simulink model "DAB"  (R2022a)
settings: Solver=ode23t  StartTime=0.0  StopTime=1.75  RelTol=1e-3
undefined symbols (not defined in the file): Ion, Lithium
libraries: spsIGBTDiodeLib x8, spsSeriesRLCBranchLib x6, spsVoltageMeasurementLib x6, spsCurrentMeasurementLib x4, spsDiodeLib x4, slpidlib x3, spsMosfetLib x2, spsBatteryLib x1, spsFuelCellStackLib x1, spsUniversalBridgeLib x1, spsLinearTransformerLib x1, spsMutualInductanceLib x1
settings Model: Creator=rahul  LastModifiedBy=DELL
settings ModelReferenceCC: EnableRefExpFcnMdlSchedulingChecks=off
settings RTWCC: Description=Generic Real-Time Target  GPUComputeCapability=5.0

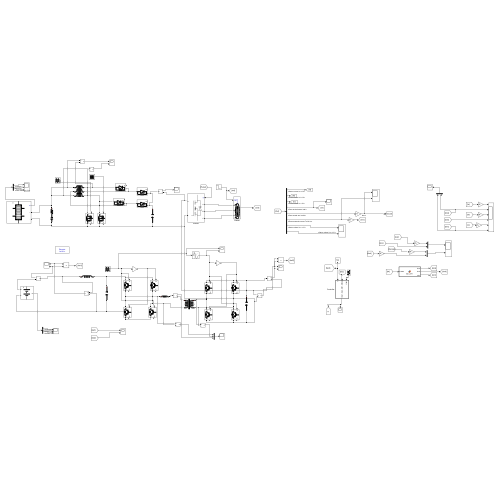
[thumbnail: Simulink's stored preview of the top-level diagram]
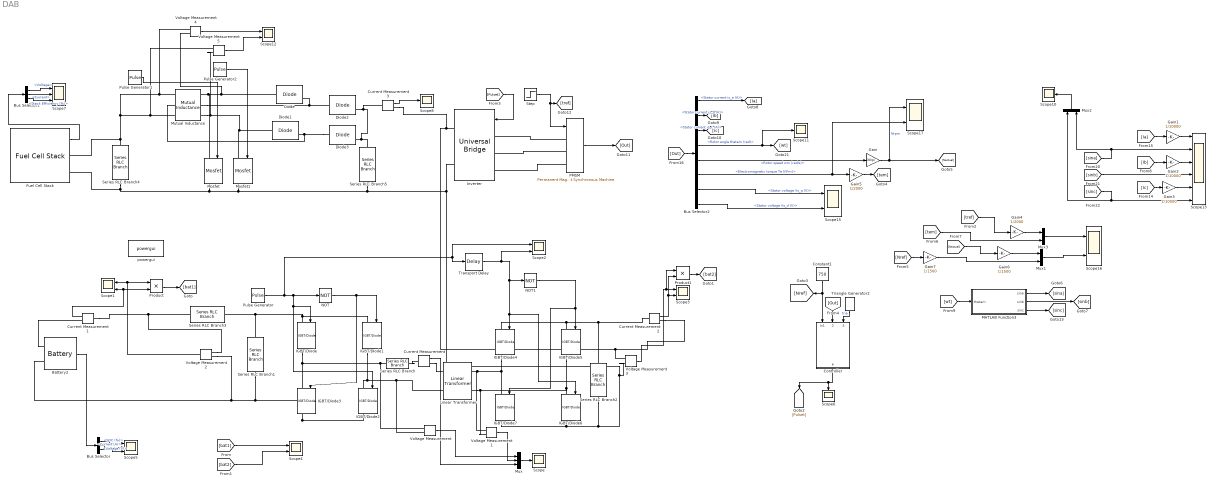
== system DAB ==
  Battery2 : spsBatteryLib/Battery  BatType=Lithium-Ion  ShowTempParam=off  ThermalPreset=no  ShowAgeParam=off  NomV=96  NomQ=26  SOC=50  Batt_Tr=30  PresetModel=on  MaxQ=26  MinV=72  FullV=111.7428  Dis_rate=11.3043  R=0.036923  Normal_OP=23.513  expZone="[103.717      1.277391]"  current=[6.5 13 32.5]  Units=Time  Tci=20  NomT=20  T2=-30  MaxQ2=4.8  FullV2=7.1  Normal_OP2=5.655  expZone2="[6.58           1]"  Rca=0.6  ti=2000  Dp=0  Neq0=0  Tsim=1e6  Ta1=25  Qeol=5.4*0.9  Reol=0.013333*1.2  Char_age=[2.3478, 3]  Dis_age=[2.3478, 10]  N1=1500  N2=10500  N3=1000  N4=1400  Ta2=45  N5=950
  Bus Selector : BusSelector  OutputSignals=SOC (%),Current (A),Voltage (V)
  Bus Selector1 : BusSelector  OutputSignals=Voltage,Current,Stack Efficiency (%)
  Bus Selector2 : BusSelector  OutputSignals=Stator current is_a (A),Stator current is_b (A),Stator current is_c (A),Rotor angle thetam (rad),Rotor speed wm (rad/s),Electromagnetic torque Te (N*m),Stator voltage Vs_q (V),Stator voltage Vs_d (V)
  Constant1 : Constant  Value=750
  Controller : Subsystem  TreatAsAtomicUnit=on
  Current Measurement{,1..3} (4 alike) : spsCurrentMeasurementLib/Current Measurement  PhasorSimulation=off  OutputType=Complex  PSBequivalent=0
  Diode{,1..3} (4 alike) : spsDiodeLib/Diode  Ron=0.001  Lon=0  Vf=0.8  IC=0  UseSnubber=0  Rs=500  Cs=250e-9  Measurements=on
  Fuel Cell Stack : spsFuelCellStackLib/Fuel Cell Stack  PresetModel=PEMFC - 6 kW - 45 Vdc  FcType=0  Detailed=Detailed  Eoc=[65,63]  NomVI=[133.3,45]  EndVI=[225,37]  Nc=65  n=55  TOp=65  AirFr=300  SuppPress=[1.5,1]  Comp=[99.95,21,1]  SignX=off  SignY=off  FlowRateH2=off  FlowRateAir=off  SystemTemp=off  SystemPH2=off  SystemPAir=off  FCDyn=off  FC_tau=1  Peak_O2=80  V_Under=10
      settings: SourceProductBaseCode=PS
  Gain : Gain  Gain=30/pi
  Gain1 : Gain  Gain=1/10000
  Gain2 : Gain  Gain=1/10000
  Gain3 : Gain  Gain=1/10000
  Gain4 : Gain  Gain=1/2000
  Gain5 : Gain  Gain=1/2000
  Gain6 : Gain  Gain=1/1500
  Gain7 : Gain  Gain=1/1500
  IGBT/Diode{,1..7} (8 alike) : spsIGBTDiodeLib/IGBT//Diode  Ron=1e-3  Rs=1e5  Cs=inf  Measurements=on
  Inverter : spsUniversalBridgeLib/Universal Bridge  Arms=3  SnubberResistance=1e5  SnubberCapacitance=inf  Device=MOSFET / Diodes  Ron=1e-3  Lon=0  ForwardVoltages="[  0  0  ]"  ForwardVoltage=0  GTOparameters=[ 10e-6 , 20e-6 ]  IGBTparameters=[ 1e-6 , 2e-6 ]  Measurements=None  Measurements_2=None  converterType=Rectifier
  Linear Transformer : spsLinearTransformerLib/Linear Transformer  UNITS=SI  NominalPower=[ 50000 20000 ]  winding1=[96 0 0]  winding2=[400 0 0]  ThreeWindings=off  winding3=[3.15e+05 0.7938 0.084225]  RmLm=[1.0804e+05 2000]  Measurements=None  DataType=on
  MATLAB Function3 : MATLAB Function  TreatAsAtomicUnit=on
  Mosfet : spsMosfetLib/Mosfet  Ron=0.1  Lon=0  Rd=0.01  Vfd=0  IC=0  Rs=1e5  Cs=inf  Measurements=on
  Mosfet1 : spsMosfetLib/Mosfet  Ron=0.1  Lon=0  Rd=0.01  Vfd=0  IC=0  Rs=1e5  Cs=inf  Measurements=on
  Mutual Inductance : spsMutualInductanceLib/Mutual Inductance  LConnTagsString=a|b|c  RConnTagsString=A|B|C  TypeOfMutual=Two or three windings with equal mutual terms  NumberOfWindings=3  SelfImpedance1=[0 2e-03]  SelfImpedance2=[0 2e-03]  ThreeWindings=on  SelfImpedance3=[0 2e-03]  MutualImpedance=[0 1.55e-03]  InductanceMatrix="[1.0 0.9  0.9 ;  0.9 1.0  0.9;  0.9 0.9 1.0 ] * 1e-3"  ResistanceMatrix="[1.0 0.9  0.9 ;  0.9 1.0  0.9;  0.9 0.9 1.0 ]"  Measurements=None
      settings: SourceProductBaseCode=PS
  Mux : Mux  Inputs=3
  Mux1 : Mux  Inputs=2
  Mux2 : Mux  Inputs=2
  Mux3 : Mux  Inputs=2
  NOT : Logic  Operator=NOT  IconShape=distinctive  AllPortsSameDT=off  OutDataTypeStr=boolean
  NOT1 : Logic  Operator=NOT  IconShape=distinctive  AllPortsSameDT=off  OutDataTypeStr=boolean
  PMSM : spsPermanentMagnetSynchronousMachineLib/Permanent Magnet Synchronous Machine  NbPhases=3  FluxDistribution=Sinusoidal  RotorType=Round  MechanicalLoad=Torque Tm  PresetModel=No  ShowDetailedParameters=on  MeasurementBus=off  Resistance=1.5  Inductance=8.5e-3  dqInductances=[0.0000094 0.000153]  La=26*10^-3  MachineConstant=Voltage Constant (V_peak L-L / krpm)  Flux=0.29634  VoltageCst=215  TorqueCst=1.778  Flat=120  Mechanical=[.00725 .0002 4 0]  PolePairs=2  InitialConditions=[0,0, 0,0]  InitialConditions5ph=[0 0 0 0 0 0]  RefAngle=90 degrees behind phase A axis (modified Park)  IterativeDiscreteModel=Trapezoidal non iterative  TsBlock=-1  TsPowergui=0
  Product : Product
  Product1 : Product
  Pulse Generator : DiscretePulseGenerator  PulseType=Time based  Period=1/(20000)  PulseWidth=60
  Pulse Generator1 : DiscretePulseGenerator  PulseType=Time based  Period=1/20000  PulseWidth=80
  Pulse Generator2 : DiscretePulseGenerator  PulseType=Time based  Period=1/20000  PulseWidth=80  PhaseDelay=1/40000
  Scope{,6,8,10..11} (5 alike) : Scope
  Scope{1..4,12,15..17} (8 alike) : Scope  NumInputPorts=2
  Scope13 : Scope  NumInputPorts=6
  Scope5 : Scope  NumInputPorts=3
  Scope7 : Scope  NumInputPorts=3
  Series RLC Branch : spsSeriesRLCBranchLib/Series RLC Branch  LConnTagsString=__new0  RConnTagsString=__new0  BranchType=L  Resistance=1  Inductance=0.02e-3  SetiL0=off  InitialCurrent=0  Capacitance=1e-6  Setx0=off  InitialVoltage=0  Measurements=None
  Series RLC Branch1 : spsSeriesRLCBranchLib/Series RLC Branch  LConnTagsString=__new0  RConnTagsString=__new0  BranchType=C  Resistance=1  Inductance=1e-3  SetiL0=off  InitialCurrent=0  Capacitance=1200e-6  Setx0=off  InitialVoltage=0  Measurements=None
  Series RLC Branch2 : spsSeriesRLCBranchLib/Series RLC Branch  LConnTagsString=__new0  RConnTagsString=__new0  BranchType=C  Resistance=1  Inductance=1e-3  SetiL0=off  InitialCurrent=0  Capacitance=1200e-6  Setx0=off  InitialVoltage=0  Measurements=None
  Series RLC Branch3 : spsSeriesRLCBranchLib/Series RLC Branch  LConnTagsString=__new0  RConnTagsString=__new0  BranchType=L  Resistance=1  Inductance=1e-3  SetiL0=off  InitialCurrent=0  Capacitance=1000e-6  Setx0=off  InitialVoltage=0  Measurements=None
  Series RLC Branch4 : spsSeriesRLCBranchLib/Series RLC Branch  LConnTagsString=__new0  RConnTagsString=__new0  BranchType=RC  Resistance=1  Inductance=1e-3  SetiL0=off  InitialCurrent=0  Capacitance=2.2e-6  Setx0=off  InitialVoltage=0  Measurements=None
  Series RLC Branch5 : spsSeriesRLCBranchLib/Series RLC Branch  LConnTagsString=__new0  RConnTagsString=__new0  BranchType=C  Resistance=1  Inductance=1e-3  SetiL0=off  InitialCurrent=0  Capacitance=750e-8  Setx0=off  InitialVoltage=0  Measurements=None
  Step : Step  Before=10  After=-10  SampleTime=0
  Transport Delay : TransportDelay  DelayTime=(1/20000)*(60/360)
  Triangle Generator2 : spsTriangleGeneratorLib/Triangle Generator  Freq=10000  Phase=90  Ts=0
  Voltage Measurement{,1..5} (6 alike) : spsVoltageMeasurementLib/Voltage Measurement  PhasorSimulation=off  OutputType=Complex  PSBequivalent=0
  powergui : spspowerguiLib/powergui  Priority=1  SimulationMode=Discrete  SampleTime=1e-6  frequency=60  Iterations=50  frequencyindice=0  Pbase=100e6  ErrMax=1e-4  UnitsV=kV  UnitsW=MW  buscounter=0  FunctionMessages=off  echomessages=off  EnableUseOfTLC=off  CurrentSourceSwitches=off  DisableSnubberDevices=off  DisableRonSwitches=off  DisableVfSwitches=off  DisplayEquations=off  AutomaticDiscreteSolvers=off  SolverType=Tustin/Backward Euler (TBE)  Interpol=off  ExternalGateDelay=off  methode=off  Ts=100  x0status=blocks  SPID=on  SwTol=0  HookPort=off  NonlinearTolerance=1e-4  nMaxIteration=100  ContinueOnMaxIteration=off  RestoreLinks=warning  ResistiveCurrentMeasurement=off  Frange=[0:2:500]  Ylog=off  Xlog=on  ShowGrid=off  save=off  variable=ZData  structure=0  ZoomFFT=off  StartTime=0.0  cycles=1  DisplayStyle=1  fundamental=60  FreqAxis=off  MaxFrequency=1000  frequencyindicesteady=1  RmsSteady=1  display=off
  wires:
  Voltage Measurement/1 -> Mux/1
  Voltage Measurement1/1 -> Mux/2
  Current Measurement/1 -> Mux/3
  Mux/1 -> Scope/1
  Pulse Generator/1 -> Transport Delay/1, Scope2/1, NOT/1, IGBT/Diode/1, IGBT/Diode2/1
  NOT/1 -> IGBT/Diode3/1, IGBT/Diode1/1
  Transport Delay/1 -> Scope2/2, NOT1/1, IGBT/Diode6/1, IGBT/Diode4/1
  NOT1/1 -> IGBT/Diode7/1, IGBT/Diode5/1
  Current Measurement1/1 -> Product/2, Scope1/2
  Voltage Measurement2/1 -> Scope1/1, Product/1
  Current Measurement2/1 -> Product1/2, Scope3/2
  Voltage Measurement3/1 -> Product1/1, Scope3/1
  Product/1 -> [bat1]
  Product1/1 -> [bat2]
  [bat1] -> Scope4/1
  [bat2] -> Scope4/2
  Battery2/1 -> Bus Selector/1
  Bus Selector/1 -> Scope5/1  "<SOC (%)>"
  Bus Selector/2 -> Scope5/2  "<Current (A)>"
  Bus Selector/3 -> Scope5/3  "<Voltage (V)>"
  Triangle Generator2/1 -> Controller/3(Inport1)  "tria"
  Controller/1(P) -> [Pulset], Scope6/1
  PMSM/1 -> [Out]
  Constant1/1 -> [Nref], Controller/1(In1)
  Step/1 -> PMSM/1, [tref]
  [Out] -> Controller/2(Inport)
  [Pulset] -> Inverter/1
  Fuel Cell Stack/1 -> Bus Selector1/1
  Bus Selector1/2 -> Scope7/2  "<Current>"
  Bus Selector1/3 -> Scope7/3  "<Stack Efficiency (%)>"
  Pulse Generator1/1 -> Mosfet/1
  Pulse Generator2/1 -> Mosfet1/1
  Current Measurement3/1 -> Scope8/1
  Bus Selector1/1 -> Scope7/1  "<Voltage>"
  Mux2/1 -> Scope10/1
  Mux3/1 -> Scope16/1
  Mux1/1 -> Scope16/2
  Gain7/1 -> Mux1/2
  [Nref] -> Gain7/1
  Gain6/1 -> Mux1/1
  [Nactual] -> Gain6/1
  [tem] -> Mux3/2
  Gain5/1 -> [tem]
  Gain4/1 -> Mux3/1
  Bus Selector2/8 -> Scope15/2  "<Stator voltage Vs_d (V)>"
  Bus Selector2/7 -> Scope15/1  "<Stator voltage Vs_q (V)>"
  Gain3/1 -> Scope13/5
  Gain2/1 -> Scope13/3
  Gain1/1 -> Scope13/1
  [sinc] -> Mux2/2, Scope13/6
  [sinb] -> Scope13/4
  [sina] -> Mux2/1, Scope13/2
  Bus Selector2/2 -> [Ib]  "<Stator current is_b (A)>"
  Bus Selector2/3 -> [Ic]  "<Stator current is_c (A)>"
  [Ib] -> Gain2/1
  [Ia] -> Gain1/1
  [Ic] -> Gain3/1
  [Out] -> Bus Selector2/1
  Bus Selector2/1 -> [Ia]  "<Stator current is_a (A)>"
  Gain/1 -> Scope17/1, [Nactual]  "Nrpm"
  Bus Selector2/5 -> Gain/1  "<Rotor speed wm (rad/s)>"
  Bus Selector2/4 -> Scope11/1, [wt]  "<Rotor angle thetam (rad)>"
  Bus Selector2/6 -> Scope17/2, Gain5/1  "<Electromagnetic torque Te (N*m)>"
  [wt] -> MATLAB Function3/1(thetam)
  MATLAB Function3/2(sinb) -> [sinb]
  MATLAB Function3/3(sinc) -> [sinc]
  MATLAB Function3/1(sina) -> [sina]
  [tref] -> Gain4/1
  Voltage Measurement4/1 -> Scope12/1
  Voltage Measurement5/1 -> Scope12/2
  connections:
  IGBT/Diode1/RConn1 -- Voltage Measurement/LConn2 -- Linear Transformer/LConn2 -- IGBT/Diode2/LConn1
  IGBT/Diode/RConn1 -- Voltage Measurement/LConn1 -- Series RLC Branch/LConn1 -- IGBT/Diode3/LConn1
  Series RLC Branch1/RConn1 -- IGBT/Diode2/RConn1 -- IGBT/Diode3/RConn1 -- Battery2/LConn2 -- Voltage Measurement2/LConn2
  IGBT/Diode5/RConn1 -- Voltage Measurement1/LConn2 -- Linear Transformer/RConn2 -- IGBT/Diode6/LConn1
  IGBT/Diode4/RConn1 -- Voltage Measurement1/LConn1 -- Linear Transformer/RConn1 -- IGBT/Diode7/LConn1
  Series RLC Branch5/RConn1 -- Mosfet/RConn1 -- Series RLC Branch4/RConn1 -- Fuel Cell Stack/RConn2 -- Mosfet1/RConn1 -- Inverter/RConn2 -- Voltage Measurement3/LConn2 -- IGBT/Diode7/RConn1 -- IGBT/Diode6/RConn1 -- Series RLC Branch2/RConn1
  Series RLC Branch/RConn1 -- Current Measurement/LConn1
  Current Measurement/RConn1 -- Linear Transformer/LConn1
  Current Measurement1/LConn1 -- Series RLC Branch3/LConn1 -- Voltage Measurement2/LConn1
  Current Measurement1/RConn1 -- Battery2/LConn1
  Series RLC Branch1/LConn1 -- IGBT/Diode/LConn1 -- IGBT/Diode1/LConn1 -- Series RLC Branch3/RConn1
  PMSM/LConn1 -- Inverter/LConn1
  PMSM/LConn2 -- Inverter/LConn2
  Current Measurement3/RConn1 -- Current Measurement2/RConn1 -- Voltage Measurement3/LConn1 -- Inverter/RConn1
  PMSM/LConn3 -- Inverter/LConn3
  IGBT/Diode4/LConn1 -- Current Measurement2/LConn1 -- Series RLC Branch2/LConn1 -- IGBT/Diode5/LConn1
  Mutual Inductance/RConn2 -- Diode/RConn1 -- Diode2/LConn1
  Mutual Inductance/LConn3 -- Voltage Measurement5/LConn1 -- Voltage Measurement4/LConn1 -- Mutual Inductance/LConn1 -- Fuel Cell Stack/RConn1 -- Series RLC Branch4/LConn1
  Mutual Inductance/RConn3 -- Voltage Measurement5/LConn2 -- Diode1/LConn1 -- Mosfet1/LConn1
  Diode/LConn1 -- Voltage Measurement4/LConn2 -- Mutual Inductance/RConn1 -- Mosfet/LConn1
  Diode3/LConn1 -- Mutual Inductance/LConn2 -- Diode1/RConn1
  Diode2/RConn1 -- Series RLC Branch5/LConn1 -- Diode3/RConn1 -- Current Measurement3/LConn1

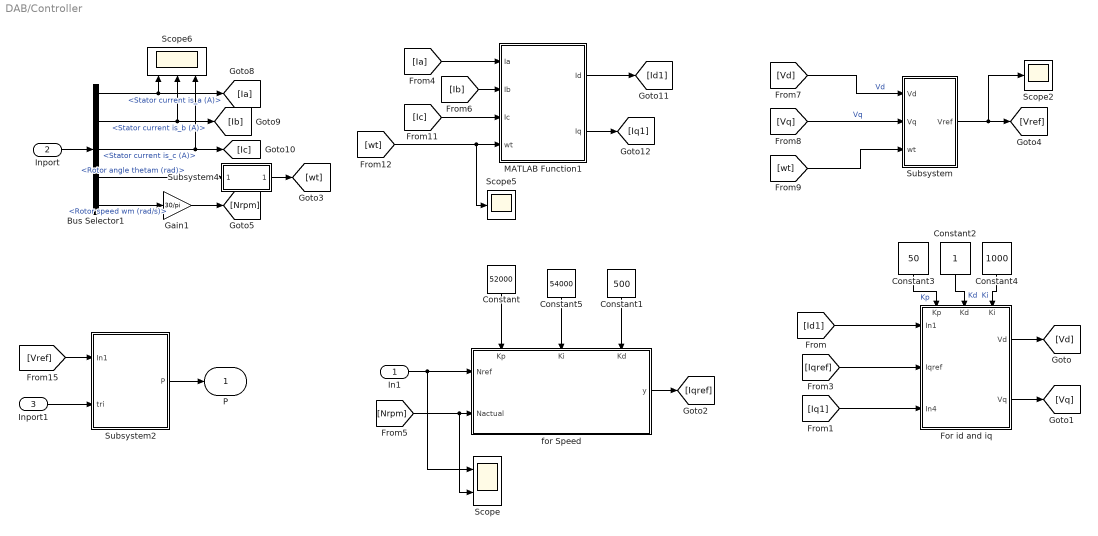
== system DAB/Controller ==
  In1 : Inport
  Inport : Inport  Port=2
  Inport1 : Inport  Port=3
  Bus Selector1 : BusSelector  OutputSignals=Stator current is_a (A),Stator current is_b (A),Stator current is_c (A),Rotor angle thetam (rad),Rotor speed wm (rad/s)
  Constant : Constant  Value=52000
  Constant1 : Constant  Value=500
  Constant2 : Constant
  Constant3 : Constant  Value=50
  Constant4 : Constant  Value=1000
  Constant5 : Constant  Value=54000
  For id and iq : Subsystem
      settings: PortSchema="{\"entries\":[{\"content\":{\"sides\":[{\"content\":{\"connectorIds\":[\"In1\",\"In2\",\"In3\"]},\"type\":\"ConnectorPlacement.EquallySpacedRectSide\",\"uuid\":\"39d41a62-c909-42e2-8909-4f5753ca638b\"},{\"content\":{\"connectorIds\":[\"Out1\",\"Out2\"],\"side\":\"RIGHT\"},\"type\":\"ConnectorPlacement.EquallySpacedRectSide\",\"uuid\":\"97cda8da-9af1-4d97-bea8-6f20bb123555\"},{\"content\":{\"connectorIds\":[\"In4\",\"In5\",\"In6\"],\"side\":\"TOP\"},\"type\":\"ConnectorPlacement.EquallySpacedRectSide\",\"uuid\":\"2e00cf8d-c3db-4fec-9118-c20b9126c3fd\"}]},\"type\":\"ConnectorPlacement.EquallySpacedConnector\",\"uuid\":\"55298a9a-772e-49ed-8058-cae6c84d6d2a\"}],\"packageUris\":[\"http://schema.mathworks.com/mf0/Connector/R2020b\"],\"version\":\"1.0\"}"
  Gain1 : Gain  Gain=30/pi
  MATLAB Function1 : MATLAB Function  TreatAsAtomicUnit=on
  Scope : Scope  NumInputPorts=2
  Scope2 : Scope
  Scope5 : Scope
  Scope6 : Scope  NumInputPorts=3
  Subsystem : Subsystem
  Subsystem2 : Subsystem
  Subsystem4 : Subsystem
  for Speed : Subsystem
      settings: PortSchema="{\"entries\":[{\"content\":{\"sides\":[{\"content\":{\"connectorIds\":[\"In1\",\"In2\"]},\"type\":\"ConnectorPlacement.EquallySpacedRectSide\",\"uuid\":\"f3063666-eb51-4108-9457-4d56db964460\"},{\"content\":{\"connectorIds\":[\"Out1\"],\"side\":\"RIGHT\"},\"type\":\"ConnectorPlacement.EquallySpacedRectSide\",\"uuid\":\"9d4387d1-2762-403b-a6f2-1844b7e47dba\"},{\"content\":{\"connectorIds\":[\"In3\",\"In4\",\"In5\"],\"side\":\"TOP\"},\"type\":\"ConnectorPlacement.EquallySpacedRectSide\",\"uuid\":\"11c44a25-b98c-459b-bb62-298add226b06\"}]},\"type\":\"ConnectorPlacement.EquallySpacedConnector\",\"uuid\":\"a132996f-a1ce-4ea7-ba38-3ba068df89dd\"}],\"packageUris\":[\"http://schema.mathworks.com/mf0/Connector/R2020b\"],\"version\":\"1.0\"}"
  P : Outport
  wires:
  Subsystem4/1(Out1) -> [wt]
  For id and iq/2(Vq) -> [Vq]
  MATLAB Function1/2(Iq) -> [Iq1]
  [wt] -> Subsystem/3(wt)
  [Id1] -> For id and iq/1(In1)
  Constant5/1 -> for Speed/4(Ki)
  [Iq1] -> For id and iq/3(In4)
  For id and iq/1(Vd) -> [Vd]
  Gain1/1 -> [Nrpm]
  Bus Selector1/1 -> [Ia], Scope6/1  "<Stator current is_a (A)>"
  MATLAB Function1/1(Id) -> [Id1]
  [Vd] -> Subsystem/1(Vd)  "Vd"
  Constant2/1 -> For id and iq/5(Kd)  "Kd"
  Bus Selector1/4 -> Subsystem4/1(<Rotor angle thetam (rad)>)  "<Rotor angle thetam (rad)>"
  Subsystem/1(Vref) -> Scope2/1, [Vref]
  Bus Selector1/2 -> [Ib], Scope6/2  "<Stator current is_b (A)>"
  Constant3/1 -> For id and iq/4(Kp)  "Kp"
  [wt] -> MATLAB Function1/4(wt), Scope5/1
  Inport/1 -> Bus Selector1/1
  In1/1 -> Scope/1, for Speed/1(Nref)
  [Vq] -> Subsystem/2(Vq)  "Vq"
  for Speed/1(y) -> [Iqref]
  Constant/1 -> for Speed/3(Kp)
  [Ia] -> MATLAB Function1/1(Ia)
  Constant4/1 -> For id and iq/6(Ki)  "Ki"
  Bus Selector1/5 -> Gain1/1  "<Rotor speed wm (rad/s)>"
  Bus Selector1/3 -> Scope6/3, [Ic]  "<Stator current is_c (A)>"
  [Iqref] -> For id and iq/2(Iqref)
  [Nrpm] -> Scope/2, for Speed/2(Nactual)
  [Ic] -> MATLAB Function1/3(Ic)
  [Ib] -> MATLAB Function1/2(Ib)
  Subsystem2/1(P) -> P/1
  [Vref] -> Subsystem2/1(In1)
  Inport1/1 -> Subsystem2/2(tri)
  Constant1/1 -> for Speed/5(Kd)

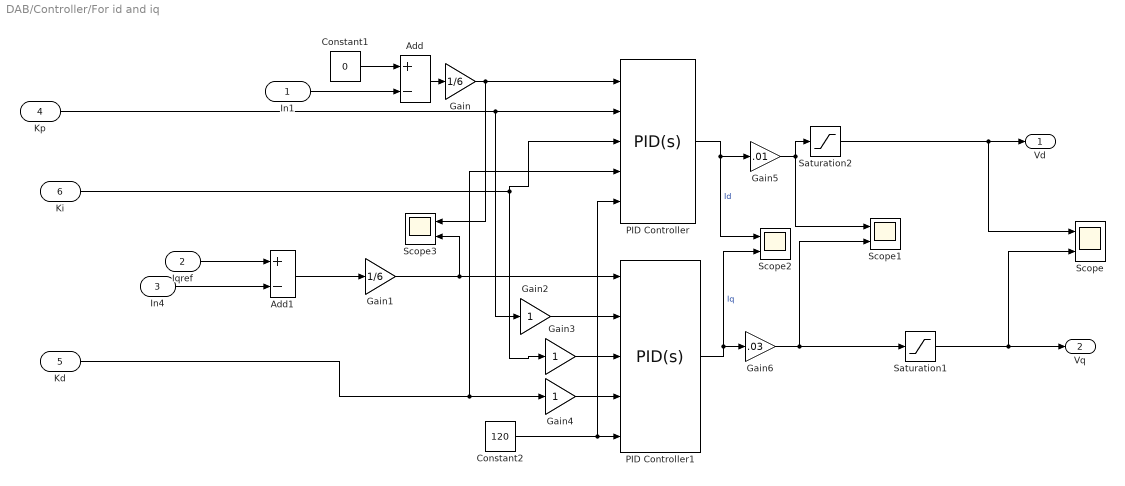
== system DAB/Controller/For id and iq ==
  In1 : Inport
  Iqref : Inport  Port=2
  In4 : Inport  Port=3
  Kp : Inport  Port=4
  Kd : Inport  Port=5
  Ki : Inport  Port=6
  Add : Sum  Inputs=+-
  Add1 : Sum  Inputs=+-
  Constant1 : Constant  Value=0
  Constant2 : Constant  Value=120
  Gain : Gain  Gain=1/6
  Gain1 : Gain  Gain=1/6
  Gain2 : Gain
  Gain3 : Gain
  Gain4 : Gain
  Gain5 : Gain  Gain=.01
  Gain6 : Gain  Gain=.03
  PID Controller : slpidlib/PID Controller  Controller=PID  Form=Parallel  TimeDomain=Continuous-time  UseExternalTs=off  SampleTime=-1  IntegratorMethod=Forward Euler  FilterMethod=Forward Euler  ControllerParametersSource=external  P=.8*10^-3  I=.5  UseKiTs=off  D=1  N=100  UseFilter=on  TunerSelectOption=Transfer Function Based (PID Tuner App)  InitialConditionSource=internal  InitialConditionForIntegrator=0  InitialConditionForFilter=0  DifferentiatorICPrevScaledInput=0  ExternalReset=none  TrackingMode=off  Kt=1  LimitOutput=off  SatLimitsSource=internal  UpperSaturationLimit=inf  LowerSaturationLimit=-inf  LinearizeAsGain=on  AntiWindupMode=none  Kb=1  POutMin=[]  POutMax=[]  IOutMin=[]  IOutMax=[]  DOutMin=[]  DOutMax=[]  NOutMin=[]  NOutMax=[]  SumOutMin=[]  SumOutMax=[]  SaturationOutMin=[]  SaturationOutMax=[]  PParamMin=[]  PParamMax=[]  IParamMin=[]  IParamMax=[]  DParamMin=[]  DParamMax=[]  NParamMin=[]  NParamMax=[]  KbParamMin=[]  KbParamMax=[]  KtParamMin=[]  KtParamMax=[]  KbOutMin=[]  KbOutMax=[]  KtOutMin=[]  KtOutMax=[]  IntegratorOutMin=[]  IntegratorOutMax=[]  FilterOutMin=[]  FilterOutMax=[]  SumI1OutMin=[]  SumI1OutMax=[]  SumI2OutMin=[]  SumI2OutMax=[]  SumI3OutMin=[]  SumI3OutMax=[]  SumI4OutMin=[]  SumI4OutMax=[]  SumDOutMin=[]  SumDOutMax=[]  DifferentiatorOutMin=[]  DifferentiatorOutMax=[]  FilterDiffOutCoefMin=[]  FilterDiffOutCoefMax=[]  ReciprocalOutMin=[]  ReciprocalOutMax=[]  SumDenOutMin=[]  SumDenOutMax=[]  SumNumOutMin=[]  SumNumOutMax=[]  DivideOutMin=[]  DivideOutMax=[]  UdiffTsProdOutMin=[]  UdiffTsProdOutMax=[]  NTsProdOutMin=[]  NTsProdOutMax=[]  UintegralTsProdOutMin=[]  UintegralTsProdOutMax=[]  UngainTsProdOutMin=[]  UngainTsProdOutMax=[]  IntegratorContinuousStateAttributes=''  IntegratorStateMustResolveToSignalObject=off  IntegratorRTWStateStorageClass=Auto  FilterContinuousStateAttributes=''  FilterStateMustResolveToSignalObject=off  FilterRTWStateStorageClass=Auto  ParallelPVariant=ExternalParameters  IdealPVariant=Disabled  IVariant=ExternalParameters  DVariant=ExternalParameters  IntegratorVariant=Continuous  SatVariant=Disabled  AWVariant=Passthrough  PCopyVariant=Disabled  TRVariant=Disabled  FdbkBlocksVariant=Forward  IdealPFdbkVariant=Disabled  SatFdbkVariant=Disabled  DerivativeFilterVariant=ContFilter  NVariant=ExternalParameters  NCopyVariant=Disabled  FilterICVariant=InternalICsFilter  IntegratorICVariant=InternalICs  ExternalResetVariant=Disabled  TRSumVariant=Passthrough  SumFdbkVariant=Disabled  SumVariant=Sum_PID  TsampFilterVariant=InternalTs  TsampNgainVariant=Passthrough  TsampIntegralVariant=Passthrough  ExternalSaturationOutDataTypeStr=Inherit: Same as second input  aMode=0
  PID Controller1 : slpidlib/PID Controller  Controller=PID  Form=Parallel  TimeDomain=Continuous-time  UseExternalTs=off  SampleTime=-1  IntegratorMethod=Forward Euler  FilterMethod=Forward Euler  ControllerParametersSource=external  P=.8*10^-3  I=.5  UseKiTs=off  D=1  N=100  UseFilter=on  TunerSelectOption=Transfer Function Based (PID Tuner App)  InitialConditionSource=internal  InitialConditionForIntegrator=0  InitialConditionForFilter=0  DifferentiatorICPrevScaledInput=0  ExternalReset=none  TrackingMode=off  Kt=1  LimitOutput=off  SatLimitsSource=internal  UpperSaturationLimit=inf  LowerSaturationLimit=-inf  LinearizeAsGain=on  AntiWindupMode=none  Kb=1  POutMin=[]  POutMax=[]  IOutMin=[]  IOutMax=[]  DOutMin=[]  DOutMax=[]  NOutMin=[]  NOutMax=[]  SumOutMin=[]  SumOutMax=[]  SaturationOutMin=[]  SaturationOutMax=[]  PParamMin=[]  PParamMax=[]  IParamMin=[]  IParamMax=[]  DParamMin=[]  DParamMax=[]  NParamMin=[]  NParamMax=[]  KbParamMin=[]  KbParamMax=[]  KtParamMin=[]  KtParamMax=[]  KbOutMin=[]  KbOutMax=[]  KtOutMin=[]  KtOutMax=[]  IntegratorOutMin=[]  IntegratorOutMax=[]  FilterOutMin=[]  FilterOutMax=[]  SumI1OutMin=[]  SumI1OutMax=[]  SumI2OutMin=[]  SumI2OutMax=[]  SumI3OutMin=[]  SumI3OutMax=[]  SumI4OutMin=[]  SumI4OutMax=[]  SumDOutMin=[]  SumDOutMax=[]  DifferentiatorOutMin=[]  DifferentiatorOutMax=[]  FilterDiffOutCoefMin=[]  FilterDiffOutCoefMax=[]  ReciprocalOutMin=[]  ReciprocalOutMax=[]  SumDenOutMin=[]  SumDenOutMax=[]  SumNumOutMin=[]  SumNumOutMax=[]  DivideOutMin=[]  DivideOutMax=[]  UdiffTsProdOutMin=[]  UdiffTsProdOutMax=[]  NTsProdOutMin=[]  NTsProdOutMax=[]  UintegralTsProdOutMin=[]  UintegralTsProdOutMax=[]  UngainTsProdOutMin=[]  UngainTsProdOutMax=[]  IntegratorContinuousStateAttributes=''  IntegratorStateMustResolveToSignalObject=off  IntegratorRTWStateStorageClass=Auto  FilterContinuousStateAttributes=''  FilterStateMustResolveToSignalObject=off  FilterRTWStateStorageClass=Auto  ParallelPVariant=ExternalParameters  IdealPVariant=Disabled  IVariant=ExternalParameters  DVariant=ExternalParameters  IntegratorVariant=Continuous  SatVariant=Disabled  AWVariant=Passthrough  PCopyVariant=Disabled  TRVariant=Disabled  FdbkBlocksVariant=Forward  IdealPFdbkVariant=Disabled  SatFdbkVariant=Disabled  DerivativeFilterVariant=ContFilter  NVariant=ExternalParameters  NCopyVariant=Disabled  FilterICVariant=InternalICsFilter  IntegratorICVariant=InternalICs  ExternalResetVariant=Disabled  TRSumVariant=Passthrough  SumFdbkVariant=Disabled  SumVariant=Sum_PID  TsampFilterVariant=InternalTs  TsampNgainVariant=Passthrough  TsampIntegralVariant=Passthrough  ExternalSaturationOutDataTypeStr=Inherit: Same as second input  aMode=0
  Saturation1 : Saturate  UpperLimit=1  LowerLimit=-1
  Saturation2 : Saturate  UpperLimit=1  LowerLimit=-1
  Scope{,1..3} (4 alike) : Scope  NumInputPorts=2
  Vd : Outport
  Vq : Outport  Port=2
  wires:
  Add/1 -> Gain/1
  Constant1/1 -> Add/1
  PID Controller1/1 -> Gain6/1, Scope2/2  "Iq"
  PID Controller/1 -> Gain5/1, Scope2/1  "Id"
  Add1/1 -> Gain1/1
  In4/1 -> Add1/2
  In1/1 -> Add/2
  Iqref/1 -> Add1/1
  Constant2/1 -> PID Controller/5, PID Controller1/5
  Kd/1 -> Gain4/1, PID Controller/4
  Kp/1 -> PID Controller/2, Gain2/1
  Gain2/1 -> PID Controller1/2
  Ki/1 -> Gain3/1, PID Controller/3
  Saturation2/1 -> Scope/1, Vd/1
  Saturation1/1 -> Scope/2, Vq/1
  Gain3/1 -> PID Controller1/3
  Gain4/1 -> PID Controller1/4
  Gain/1 -> PID Controller/1, Scope3/1
  Gain1/1 -> PID Controller1/1, Scope3/2
  Gain5/1 -> Saturation2/1, Scope1/1
  Gain6/1 -> Scope1/2, Saturation1/1

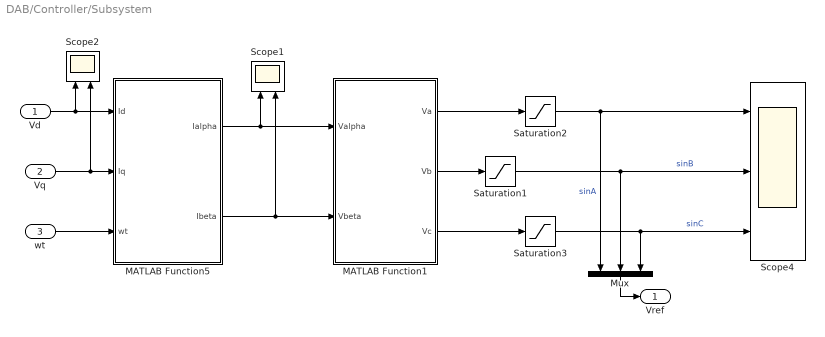
== system DAB/Controller/Subsystem ==
  Vd : Inport
  Vq : Inport  Port=2
  wt : Inport  Port=3
  MATLAB Function1 : MATLAB Function  TreatAsAtomicUnit=on
  MATLAB Function5 : MATLAB Function  TreatAsAtomicUnit=on
  Mux : Mux  Inputs=3
  Saturation1 : Saturate  UpperLimit=1  LowerLimit=-1
  Saturation2 : Saturate  UpperLimit=1  LowerLimit=-1
  Saturation3 : Saturate  UpperLimit=1  LowerLimit=-1
  Scope1 : Scope  NumInputPorts=2
  Scope2 : Scope  NumInputPorts=2
  Scope4 : Scope  NumInputPorts=3
  Vref : Outport
  wires:
  MATLAB Function1/1(Va) -> Saturation2/1
  MATLAB Function1/3(Vc) -> Saturation3/1
  Vq/1 -> MATLAB Function5/2(Iq), Scope2/2
  Vd/1 -> MATLAB Function5/1(Id), Scope2/1
  wt/1 -> MATLAB Function5/3(wt)
  MATLAB Function1/2(Vb) -> Saturation1/1
  Mux/1 -> Vref/1
  MATLAB Function5/1(Ialpha) -> MATLAB Function1/1(Valpha), Scope1/1
  MATLAB Function5/2(Ibeta) -> MATLAB Function1/2(Vbeta), Scope1/2
  Saturation2/1 -> Scope4/1, Mux/1  "sinA"
  Saturation1/1 -> Scope4/2, Mux/2  "sinB"
  Saturation3/1 -> Scope4/3, Mux/3  "sinC"

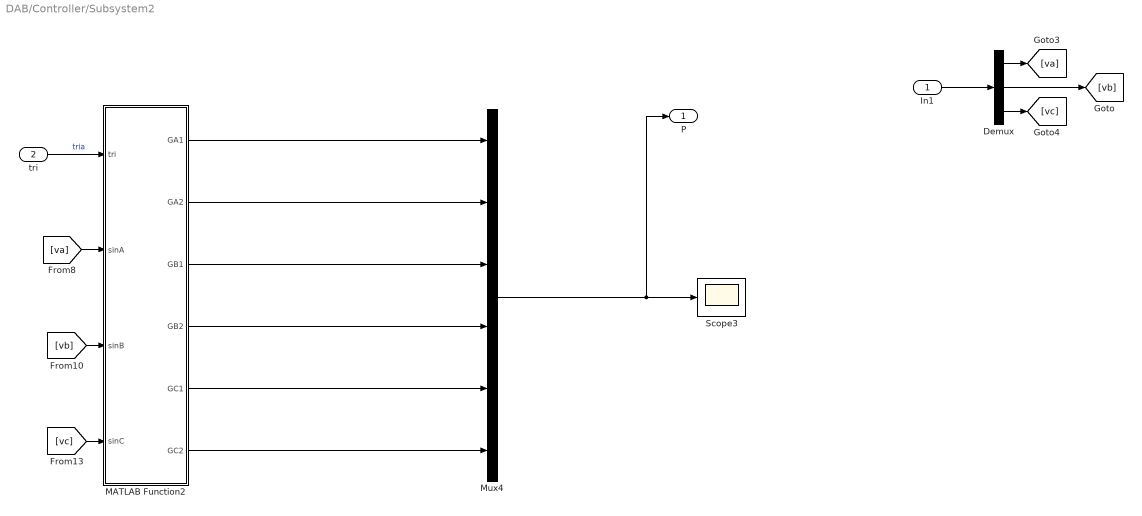
== system DAB/Controller/Subsystem2 ==
  In1 : Inport
  tri : Inport  Port=2
  Demux : Demux  Outputs=3
  MATLAB Function2 : MATLAB Function  TreatAsAtomicUnit=on
  Mux4 : Mux  Inputs=6
  Scope3 : Scope
  P : Outport
  wires:
  [vc] -> MATLAB Function2/4(sinC)
  [vb] -> MATLAB Function2/3(sinB)
  Mux4/1 -> P/1, Scope3/1
  [va] -> MATLAB Function2/2(sinA)
  In1/1 -> Demux/1
  Demux/1 -> [va]
  Demux/3 -> [vc]
  Demux/2 -> [vb]
  tri/1 -> MATLAB Function2/1(tri)  "tria"
  MATLAB Function2/1(GA1) -> Mux4/1
  MATLAB Function2/6(GC2) -> Mux4/6
  MATLAB Function2/5(GC1) -> Mux4/5
  MATLAB Function2/4(GB2) -> Mux4/4
  MATLAB Function2/3(GB1) -> Mux4/3
  MATLAB Function2/2(GA2) -> Mux4/2

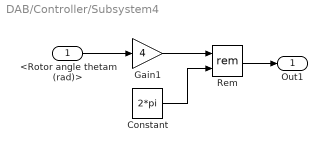
== system DAB/Controller/Subsystem4 ==
  <Rotor angle thetam (rad)> : Inport
  Constant : Constant  Value=2*pi
  Gain1 : Gain  Gain=4
  Rem : Math  Operator=rem
  Out1 : Outport
  wires:
  Constant/1 -> Rem/2
  Gain1/1 -> Rem/1
  Rem/1 -> Out1/1
  <Rotor angle thetam (rad)>/1 -> Gain1/1

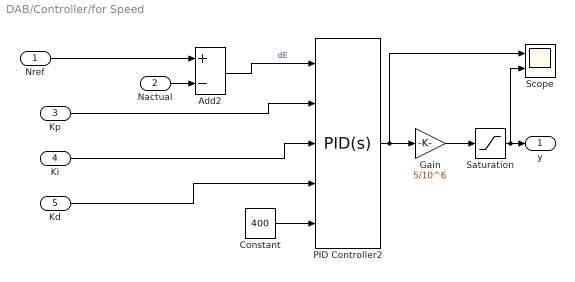
== system DAB/Controller/for Speed ==
  Nref : Inport
  Nactual : Inport  Port=2
  Kp : Inport  Port=3
  Ki : Inport  Port=4
  Kd : Inport  Port=5
  Add2 : Sum  Inputs=+-
  Constant : Constant  Value=400
  Gain : Gain  Gain=5/10^6
  PID Controller2 : slpidlib/PID Controller  Controller=PID  Form=Parallel  TimeDomain=Continuous-time  UseExternalTs=off  SampleTime=-1  IntegratorMethod=Forward Euler  FilterMethod=Forward Euler  ControllerParametersSource=external  P=.1*10^3  I=.25  UseKiTs=off  D=10  N=100  UseFilter=on  TunerSelectOption=Transfer Function Based (PID Tuner App)  ZeroCross=off  InitialConditionSource=internal  InitialConditionForIntegrator=1  InitialConditionForFilter=0  DifferentiatorICPrevScaledInput=0  ExternalReset=none  TrackingMode=off  Kt=1  LimitOutput=off  SatLimitsSource=internal  UpperSaturationLimit=inf  LowerSaturationLimit=-inf  LinearizeAsGain=on  AntiWindupMode=none  Kb=1  POutMin=[]  POutMax=[]  IOutMin=[]  IOutMax=[]  DOutMin=[]  DOutMax=[]  NOutMin=[]  NOutMax=[]  SumOutMin=[]  SumOutMax=[]  SaturationOutMin=[]  SaturationOutMax=[]  PParamMin=[]  PParamMax=[]  IParamMin=[]  IParamMax=[]  DParamMin=[]  DParamMax=[]  NParamMin=[]  NParamMax=[]  KbParamMin=[]  KbParamMax=[]  KtParamMin=[]  KtParamMax=[]  KbOutMin=[]  KbOutMax=[]  KtOutMin=[]  KtOutMax=[]  IntegratorOutMin=[]  IntegratorOutMax=[]  FilterOutMin=[]  FilterOutMax=[]  SumI1OutMin=[]  SumI1OutMax=[]  SumI2OutMin=[]  SumI2OutMax=[]  SumI3OutMin=[]  SumI3OutMax=[]  SumI4OutMin=[]  SumI4OutMax=[]  SumDOutMin=[]  SumDOutMax=[]  DifferentiatorOutMin=[]  DifferentiatorOutMax=[]  FilterDiffOutCoefMin=[]  FilterDiffOutCoefMax=[]  ReciprocalOutMin=[]  ReciprocalOutMax=[]  SumDenOutMin=[]  SumDenOutMax=[]  SumNumOutMin=[]  SumNumOutMax=[]  DivideOutMin=[]  DivideOutMax=[]  UdiffTsProdOutMin=[]  UdiffTsProdOutMax=[]  NTsProdOutMin=[]  NTsProdOutMax=[]  UintegralTsProdOutMin=[]  UintegralTsProdOutMax=[]  UngainTsProdOutMin=[]  UngainTsProdOutMax=[]  IntegratorContinuousStateAttributes=''  IntegratorStateMustResolveToSignalObject=off  IntegratorRTWStateStorageClass=Auto  FilterContinuousStateAttributes=''  FilterStateMustResolveToSignalObject=off  FilterRTWStateStorageClass=Auto  ParallelPVariant=ExternalParameters  IdealPVariant=Disabled  IVariant=ExternalParameters  DVariant=ExternalParameters  IntegratorVariant=Continuous  SatVariant=Disabled  AWVariant=Passthrough  PCopyVariant=Disabled  TRVariant=Disabled  FdbkBlocksVariant=Forward  IdealPFdbkVariant=Disabled  SatFdbkVariant=Disabled  DerivativeFilterVariant=ContFilter  NVariant=ExternalParameters  NCopyVariant=Disabled  FilterICVariant=InternalICsFilter  IntegratorICVariant=InternalICs  ExternalResetVariant=Disabled  TRSumVariant=Passthrough  SumFdbkVariant=Disabled  SumVariant=Sum_PID  TsampFilterVariant=InternalTs  TsampNgainVariant=Passthrough  TsampIntegralVariant=Passthrough  ExternalSaturationOutDataTypeStr=Inherit: Same as second input  aMode=0
  Saturation : Saturate  UpperLimit=12  LowerLimit=-12
  Scope : Scope  NumInputPorts=2
  y : Outport
  wires:
  Nactual/1 -> Add2/2
  Kp/1 -> PID Controller2/2
  Add2/1 -> PID Controller2/1  "dE"
  Ki/1 -> PID Controller2/3
  Nref/1 -> Add2/1
  PID Controller2/1 -> Scope/1, Gain/1
  Saturation/1 -> Scope/2, y/1
  Gain/1 -> Saturation/1
  Kd/1 -> PID Controller2/4
  Constant/1 -> PID Controller2/5

== matlab function DAB/MATLAB Function3 ==
  data: thetam input; sina output; sinb output; sinc output
function [sina,sinb, sinc]  = Sin_ref1(thetam)
 
    % Theta and sin cos functions

    sina = sin(4 * thetam+(pi/2));
    sinb = sin((4 * thetam+(pi/2))-(pi/1.5));
    sinc = sin((4 * thetam+(pi/2))+(pi/1.5));
   
    
end

== matlab function DAB/Controller/MATLAB Function1 ==
  data: Ia input; Id output; Ib input; Ic input; Iq output; wt input
function [Id, Iq] = ClarknPark(Ia, Ib, Ic, wt)

%%%%% Clark transform
I_abc = [Ia; Ib; Ic];

T_clark =[1, -.5, -.5; 0, sqrt(3)/2, -sqrt(3)/2];
I_alphabeta = (2/3)*T_clark* I_abc;

%%%%% Park transform
theta = (wt)-(pi/2);

%%%%%%%%%%% rotating angle is aligned 90 degrees behind Ia
T_park = [cos(theta), sin(theta); -sin(theta), cos(theta)];

I_dq = T_park* I_alphabeta;

Ial = I_alphabeta(1);
Ibl = I_alphabeta(2);

Id = I_dq(1);
Iq = I_dq(2);


end

== matlab function DAB/Controller/Subsystem/MATLAB Function1 ==
  data: Valpha input; Va output; Vbeta input; Vb output; Vc output
function [Va, Vb, Vc] = InvClarkk(Valpha, Vbeta)

%%%%% Clark transform
Valphabeta = [Valpha; Vbeta];

T_inclark =[1, 0; -.5, sqrt(3)/2; -.5, -sqrt(3)/2;];

Vabc = T_inclark* Valphabeta;

Va = Vabc(1);
Vb = Vabc(2);
Vc = Vabc(3);


end

== matlab function DAB/Controller/Subsystem/MATLAB Function5 ==
  data: Id input; Ialpha output; Iq input; Ibeta output; wt input
function [Ialpha, Ibeta] = Invpark(Id, Iq, wt)

%%%%% Clark transform
I_dq = [Id; Iq];




%%%%% Park transform
%%%%%%%%%%% rotating angle is aligned 90 degrees behind Ia
theta = (wt)-(pi/2);

T_park = [cos(theta), -sin(theta); sin(theta), cos(theta)];
I_alphabeta = T_park*I_dq;

Ialpha = I_alphabeta(1);
Ibeta = I_alphabeta(2);

end

== matlab function DAB/Controller/Subsystem2/MATLAB Function2 ==
  data: tri input; GA1 output; sinA input; sinB input; sinC input; GA2 output; GB1 output; GB2 output; GC1 output; GC2 output
function [GA1, GA2, GB1, GB2, GC1, GC2] = fcn(tri, sinA, sinB, sinC)

    %%%%%%%%%%%% Comparison for Leg A %%%%%%%%%%%
    e_a = sinA - tri;
   
    %%%%%%%%%%%% Comparison for Leg B %%%%%%%%%%%
    e_b = sinB - tri;

    %%%%%%%%%%%% Comparison for Leg C %%%%%%%%%%%
    e_c = sinC - tri;
    

    %%%%%%%%%%% Switching pulses for Leg A %%%%%%%%%%%
    if e_a >= 0
        GA1 = 1;
        GA2 = 0;
    else
        GA1 = 0;
        GA2 = 1;
    end

 

    %%%%%%%%%%% Switching pulses for Leg B %%%%%%%%%%%
    if e_b >= 0
        GB1 = 1;
        GB2 = 0;
    else
        GB1 = 0;
        GB2 = 1;
    end


    %%%%%%%%%%% Switching pulses for Leg C %%%%%%%%%%%
    if e_c >= 0
        GC1 = 1;
        GC2 = 0;
    else
        GC1 = 0;
        GC2 = 1;
    end

  

end
